simulink model "NN_MPC"  (R2018a)
settings: Solver=FixedStepAuto  SolverName=VariableStepAuto  StartTime=0.0  StopTime=40  FixedStep=0.01  RelTol=1e-3
values from neighbouring files (symbols this model uses):
  a = 0.95    [Params.mat]    (also in R_neural_function.m = 2 ./ (1 + exp(-2*n)) - 1; neural_Nc.m = 2 ./ (1 + exp(-2*n)) - 1; neural_Np.m = 2 ./ (1 + exp(-2*n)) - 1; neural_Qy.m = 2 ./ (1 + exp(-2*n)) - 1)
  Cf = 19000    [Params.mat]
  Cr = 33000    [Params.mat]
  deltau_max = 0.261799387799    [Params.mat]
  deltau_min = -0.261799387799    [Params.mat]
  dt = 0.1    [Params.mat]
  Iz = 2875    [Params.mat]
  lf = 1.2    [Params.mat]
  lr = 1.6    [Params.mat]
  m = 1575    [Params.mat]
  N = 10    [Params.mat]
  Nc = 5    [Params.mat]
  Np = 35    [Params.mat]
  Q = 5    [Params.mat]    (also in R_neural_function.m = 0; neural_Nc.m = 0; neural_Np.m = 0; neural_Qy.m = 0)
  R = 0.1    [Params.mat]
  u_max = 0.523598775598    [Params.mat]
  u_min = -0.523598775598    [Params.mat]
  y_max = 200    [Params.mat]
  y_min = -200    [Params.mat]
undefined symbols (not defined in the file or in its folder): neural_Nc, neural_Np, neural_Qy, neural_R, sigbuilder_block
libraries: autolibutils x8, autolibshared x6, vehdynlibviscommon x2, simulink x2
(part 1 of 4)
settings Model: Creator=yassine  LastModifiedBy=yassi
settings DataIOCC: ReturnWorkspaceOutputs=on
settings SFSimCC: SimUseLocalCustomCode=on
settings RTWCC: RTWUseLocalCustomCode=on

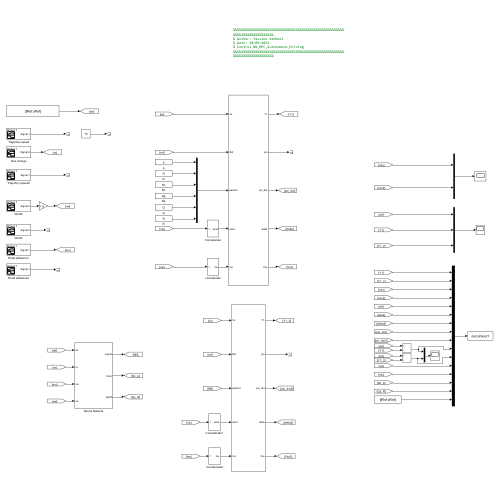
[thumbnail: Simulink's stored preview of the top-level diagram]
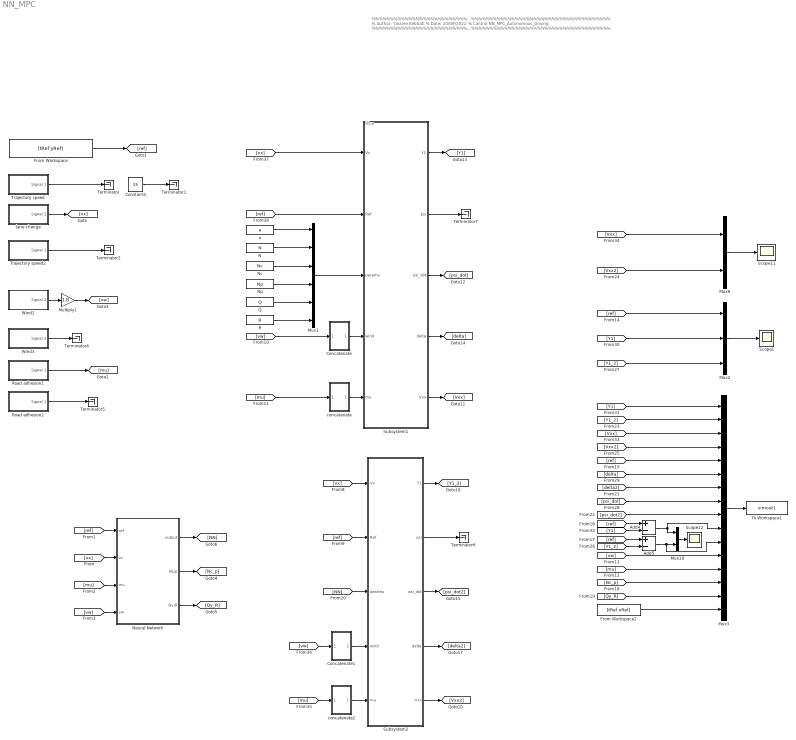
== system NN_MPC ==
  note: %%%%%%%%%%%%%%%%%%%%%%%%%%%%%%%%%%%%%%%%%%%%%%%%%%%%%%%%%%%%%%%%%%%%%%%%%%%
      | % Author: Yassine Kebbati
      | % Date: 20/09/2022
      | % Control NN_MPC_Autonomous_Driving
      | %%%%%%%%%%%%%%%%%%%%%%%%%%%%%%%%%%%%%%%%%%%%%%%%%%%%%%%%%%%%%%%%%%%%%%%%%%%
  note: Blue
  Add4 : Sum  Inputs=+-
  Add5 : Sum  Inputs=+-
  Concatenate : Subsystem
  Concatenate1 : Subsystem
  Constant4 : Constant  Value=15
  From Workspace : FromWorkspace  VariableName=[tRef yRef]
  From Workspace2 : FromWorkspace  VariableName=[tRef xRef]
  Multiply1 : Gain  Gain=1.8
  Mux1 : Mux  Inputs=6
  Mux10 : Mux  Inputs=2
  Mux2 : Mux  Inputs=3
  Mux3 : Mux  Inputs=16
  Mux9 : Mux  Inputs=2
  N : Constant  Value=N
  Nc : Constant  Value=Nc
  Neural Network : Subsystem
  Np : Constant  Value=Np
  Q : Constant  Value=Q
  R : Constant  Value=R
  Road adhesion1 : Subsystem  Tag=STV Subsys  LoadFcn=sigbuilder_block('load');  StartFcn=sigbuilder_block('start');  StopFcn=sigbuilder_block('stop');  ClipboardFcn=sigbuilder_block('clipboard');  mask(Sigbuilder block){tuvar=[0:10]}
      mask help: Simulink:masks:SigbuilderBlock_MD
      mask init:
      | if ~strcmp(get_param(bdroot(gcbh),'SimulationStatus'),'stopped') tuvar = sigbuilder_block('maskInit'); end
      settings: CopyFcn=sigbuilder_block('copy');  DeleteFcn=sigbuilder_block('delete');  ModelCloseFcn=sigbuilder_block('modelClose');  PreSaveFcn=sigbuilder_block('preSave');  PauseFcn=sigbuilder_block('pause');  ContinueFcn=sigbuilder_block('continue');  NameChangeFcn=sigbuilder_block('namechange');  OpenFcn=sigbuilder_block('open',[6 22.5 1428 689.25 ]);  CloseFcn=sigbuilder_block('close');
      mask Display: plot(0, 0, 100, 100,[2, 2, 32, 32, 2], [68, 8, 8, 68, 68],[32, 2], [38, 38], [32, 19, 2],[53, 60, 44], [32, 17, 17, 2],[16, 16, 31, 31]);txt = getActiveGroup(gcbh);text(2, 100, txt,'verticalAlignment', 'top');
  Road adhesion2 : Subsystem  Tag=STV Subsys  LoadFcn=sigbuilder_block('load');  StartFcn=sigbuilder_block('start');  StopFcn=sigbuilder_block('stop');  ClipboardFcn=sigbuilder_block('clipboard');  mask(Sigbuilder block){tuvar=[0:10]}
      mask help: Simulink:masks:SigbuilderBlock_MD
      mask init:
      | if ~strcmp(get_param(bdroot(gcbh),'SimulationStatus'),'stopped') tuvar = sigbuilder_block('maskInit'); end
      settings: CopyFcn=sigbuilder_block('copy');  DeleteFcn=sigbuilder_block('delete');  ModelCloseFcn=sigbuilder_block('modelClose');  PreSaveFcn=sigbuilder_block('preSave');  PauseFcn=sigbuilder_block('pause');  ContinueFcn=sigbuilder_block('continue');  NameChangeFcn=sigbuilder_block('namechange');  OpenFcn=sigbuilder_block('open',[1446 57 1428 689.25 ]);  CloseFcn=sigbuilder_block('close');
      mask Display: plot(0, 0, 100, 100,[2, 2, 32, 32, 2], [68, 8, 8, 68, 68],[32, 2], [38, 38], [32, 19, 2],[53, 60, 44], [32, 17, 17, 2],[16, 16, 31, 31]);txt = getActiveGroup(gcbh);text(2, 100, txt,'verticalAlignment', 'top');
  Scope1 : Scope
  Scope11 : Scope
  Scope12 : Scope
  Subsystem1 : Subsystem
  Subsystem2 : Subsystem
  Terminator{,1..2,4..7} (7 alike) : Terminator
  To Workspace1 : ToWorkspace  VariableName=simout1  SaveFormat=Timeseries  SampleTime=-1
  Trajectory speed : Subsystem  Tag=STV Subsys  LoadFcn=sigbuilder_block('load');  StartFcn=sigbuilder_block('start');  StopFcn=sigbuilder_block('stop');  ClipboardFcn=sigbuilder_block('clipboard');  mask(Sigbuilder block){tuvar=[0:10]}
      mask help: Simulink:masks:SigbuilderBlock_MD
      mask init:
      | if ~strcmp(get_param(bdroot(gcbh),'SimulationStatus'),'stopped') tuvar = sigbuilder_block('maskInit'); end
      settings: CopyFcn=sigbuilder_block('copy');  DeleteFcn=sigbuilder_block('delete');  ModelCloseFcn=sigbuilder_block('modelClose');  PreSaveFcn=sigbuilder_block('preSave');  PauseFcn=sigbuilder_block('pause');  ContinueFcn=sigbuilder_block('continue');  NameChangeFcn=sigbuilder_block('namechange');  OpenFcn=sigbuilder_block('open',[6 22.5 1428 689.25 ]);  CloseFcn=sigbuilder_block('close');
      mask Display: plot(0, 0, 100, 100,[2, 2, 32, 32, 2], [68, 8, 8, 68, 68],[32, 2], [38, 38], [32, 19, 2],[53, 60, 44], [32, 17, 17, 2],[16, 16, 31, 31]);txt = getActiveGroup(gcbh);text(2, 100, txt,'verticalAlignment', 'top');
  Trajectory speed2 : Subsystem  Tag=STV Subsys  LoadFcn=sigbuilder_block('load');  StartFcn=sigbuilder_block('start');  StopFcn=sigbuilder_block('stop');  ClipboardFcn=sigbuilder_block('clipboard');  mask(Sigbuilder block){tuvar=[0:10]}
      mask help: Simulink:masks:SigbuilderBlock_MD
      mask init:
      | if ~strcmp(get_param(bdroot(gcbh),'SimulationStatus'),'stopped') tuvar = sigbuilder_block('maskInit'); end
      settings: CopyFcn=sigbuilder_block('copy');  DeleteFcn=sigbuilder_block('delete');  ModelCloseFcn=sigbuilder_block('modelClose');  PreSaveFcn=sigbuilder_block('preSave');  PauseFcn=sigbuilder_block('pause');  ContinueFcn=sigbuilder_block('continue');  NameChangeFcn=sigbuilder_block('namechange');  OpenFcn=sigbuilder_block('open',[6 3.75 1428 648.75 ]);  CloseFcn=sigbuilder_block('close');
      mask Display: plot(0, 0, 100, 100,[2, 2, 32, 32, 2], [68, 8, 8, 68, 68],[32, 2], [38, 38], [32, 19, 2],[53, 60, 44], [32, 17, 17, 2],[16, 16, 31, 31]);txt = getActiveGroup(gcbh);text(2, 100, txt,'verticalAlignment', 'top');
  Wind2 : Subsystem  Tag=STV Subsys  LoadFcn=sigbuilder_block('load');  StartFcn=sigbuilder_block('start');  StopFcn=sigbuilder_block('stop');  ClipboardFcn=sigbuilder_block('clipboard');  mask(Sigbuilder block){tuvar=[0:10]}
      mask help: Simulink:masks:SigbuilderBlock_MD
      mask init:
      | if ~strcmp(get_param(bdroot(gcbh),'SimulationStatus'),'stopped') tuvar = sigbuilder_block('maskInit'); end
      settings: CopyFcn=sigbuilder_block('copy');  DeleteFcn=sigbuilder_block('delete');  ModelCloseFcn=sigbuilder_block('modelClose');  PreSaveFcn=sigbuilder_block('preSave');  PauseFcn=sigbuilder_block('pause');  ContinueFcn=sigbuilder_block('continue');  NameChangeFcn=sigbuilder_block('namechange');  OpenFcn=sigbuilder_block('open',[6 85.5 1428 608.25 ]);  CloseFcn=sigbuilder_block('close');
      mask Display: plot(0, 0, 100, 100,[2, 2, 32, 32, 2], [68, 8, 8, 68, 68],[32, 2], [38, 38], [32, 19, 2],[53, 60, 44], [32, 17, 17, 2],[16, 16, 31, 31]);txt = getActiveGroup(gcbh);text(2, 100, txt,'verticalAlignment', 'top');
  Wind3 : Subsystem  Tag=STV Subsys  LoadFcn=sigbuilder_block('load');  StartFcn=sigbuilder_block('start');  StopFcn=sigbuilder_block('stop');  ClipboardFcn=sigbuilder_block('clipboard');  mask(Sigbuilder block){tuvar=[0:10]}
      mask help: Simulink:masks:SigbuilderBlock_MD
      mask init:
      | if ~strcmp(get_param(bdroot(gcbh),'SimulationStatus'),'stopped') tuvar = sigbuilder_block('maskInit'); end
      settings: CopyFcn=sigbuilder_block('copy');  DeleteFcn=sigbuilder_block('delete');  ModelCloseFcn=sigbuilder_block('modelClose');  PreSaveFcn=sigbuilder_block('preSave');  PauseFcn=sigbuilder_block('pause');  ContinueFcn=sigbuilder_block('continue');  NameChangeFcn=sigbuilder_block('namechange');  OpenFcn=sigbuilder_block('open',[6 22.5 1428 689.25 ]);  CloseFcn=sigbuilder_block('close');
      mask Display: plot(0, 0, 100, 100,[2, 2, 32, 32, 2], [68, 8, 8, 68, 68],[32, 2], [38, 38], [32, 19, 2],[53, 60, 44], [32, 17, 17, 2],[16, 16, 31, 31]);txt = getActiveGroup(gcbh);text(2, 100, txt,'verticalAlignment', 'top');
  a : Constant  Value=a
  concatenate : Subsystem
  concatenate2 : Subsystem
  lane change : Subsystem  Tag=STV Subsys  LoadFcn=sigbuilder_block('load');  StartFcn=sigbuilder_block('start');  StopFcn=sigbuilder_block('stop');  ClipboardFcn=sigbuilder_block('clipboard');  mask(Sigbuilder block){tuvar=[0:10]}
      mask help: Simulink:masks:SigbuilderBlock_MD
      mask init:
      | if ~strcmp(get_param(bdroot(gcbh),'SimulationStatus'),'stopped') tuvar = sigbuilder_block('maskInit'); end
      settings: CopyFcn=sigbuilder_block('copy');  DeleteFcn=sigbuilder_block('delete');  ModelCloseFcn=sigbuilder_block('modelClose');  PreSaveFcn=sigbuilder_block('preSave');  PauseFcn=sigbuilder_block('pause');  ContinueFcn=sigbuilder_block('continue');  NameChangeFcn=sigbuilder_block('namechange');  OpenFcn=sigbuilder_block('open',[6 22.5 1428 689.25 ]);  CloseFcn=sigbuilder_block('close');
      mask Display: plot(0, 0, 100, 100,[2, 2, 32, 32, 2], [68, 8, 8, 68, 68],[32, 2], [38, 38], [32, 19, 2],[53, 60, 44], [32, 17, 17, 2],[16, 16, 31, 31]);txt = getActiveGroup(gcbh);text(2, 100, txt,'verticalAlignment', 'top');
  wires:
  Neural Network/2(Nc/p) -> [Nc_p]
  [vw] -> Neural Network/4(vw)
  [mu] -> Neural Network/3(mu)
  Neural Network/1(output) -> [NN]
  Neural Network/3(Qy/R) -> [Qy_R]
  [ref] -> Neural Network/1(ref)
  [vx] -> Neural Network/2(vx)
  Subsystem1/5(Vxx) -> [Vxx]
  Q/1 -> Mux1/5
  [Nc_p] -> Mux3/14
  Subsystem1/2(psi) -> Terminator7/1
  [vw] -> Concatenate/1(In1)
  [NN] -> Subsystem2/3(params)
  Subsystem1/4(delta) -> [delta]
  R/1 -> Mux1/6
  [Y1_2] -> Mux2/3
  [Y1] -> Add4/2
  Subsystem1/1(Y1) -> [Y1]
  Subsystem2/2(psi) -> Terminator6/1
  [psi_dot2] -> Mux3/9
  Np/1 -> Mux1/4
  [Vxx] -> Mux3/3
  [psi_dot] -> Mux3/8
  [mu] -> concatenate2/1(In1)
  lane change/1(Signal 2) -> [vx]
  Trajectory speed2/1(Signal 1) -> Terminator2/1
  [vx] -> Subsystem2/1(Vx)
  From Workspace/1 -> [ref]
  [Qy_R] -> Mux3/15
  Road adhesion2/1(Signal 1) -> Terminator5/1
  concatenate/1(mu) -> Subsystem1/5(mu)
  Mux9/1 -> Scope11/1
  Wind2/1(Signal 2) -> Multiply1/1
  From Workspace2/1 -> Mux3/16
  Add4/1 -> Mux3/10, Mux10/1
  Trajectory speed/1(Signal 1) -> Terminator/1
  [ref] -> Add5/1
  [ref] -> Subsystem1/2("Ref ")
  Concatenate1/1(wind) -> Subsystem2/4(wind)
  [ref] -> Subsystem2/2("Ref ")
  [vw] -> Concatenate1/1(In1)
  [Y1] -> Mux2/2
  Add5/1 -> Mux3/11, Mux10/2
  [delta] -> Mux3/6
  Nc/1 -> Mux1/3
  [Y1_2] -> Add5/2
  [Vxx2] -> Mux9/2
  Mux3/1 -> To Workspace1/1
  Mux2/1 -> Scope1/1
  Concatenate/1(wind) -> Subsystem1/4(wind)
  [Y1_2] -> Mux3/2
  [Vxx2] -> Mux3/4
  Subsystem1/3(psi_dot) -> [psi_dot]
  Subsystem2/1(Y1) -> [Y1_2]
  Wind3/1(Signal 2) -> Terminator4/1
  Subsystem2/5(Vxx) -> [Vxx2]
  [delta2] -> Mux3/7
  [ref] -> Mux3/5
  Subsystem2/4(delta) -> [delta2]
  Mux1/1 -> Subsystem1/3(params)
  Multiply1/1 -> [vw]
  Road adhesion1/1(Signal 1) -> [mu]
  Constant4/1 -> Terminator1/1
  [Vxx] -> Mux9/1
  Mux10/1 -> Scope12/1
  [ref] -> Mux2/1
  concatenate2/1(mu) -> Subsystem2/5(mu)
  [mu] -> Mux3/13
  [mu] -> concatenate/1(In1)
  [Y1] -> Mux3/1
  [vw] -> Mux3/12
  Subsystem2/3(psi_dot) -> [psi_dot2]
  [vx] -> Subsystem1/1(Vx)
  N/1 -> Mux1/2
  a/1 -> Mux1/1
  [ref] -> Add4/1

== system NN_MPC/Concatenate ==
  In1 : Inport
  Constant1 : Constant  Value=0
  Matrix Concatenate : Concatenate  NumInputs=3  Mode=Multidimensional array  ConcatenateDimension=2
  wind : Outport
  wires:
  Constant1/1 -> Matrix Concatenate/3, Matrix Concatenate/1
  In1/1 -> Matrix Concatenate/2
  Matrix Concatenate/1 -> wind/1

== system NN_MPC/Concatenate1 ==
  In1 : Inport
  Constant1 : Constant  Value=0
  Matrix Concatenate : Concatenate  NumInputs=3  Mode=Multidimensional array  ConcatenateDimension=2
  wind : Outport
  wires:
  Constant1/1 -> Matrix Concatenate/3, Matrix Concatenate/1
  In1/1 -> Matrix Concatenate/2
  Matrix Concatenate/1 -> wind/1

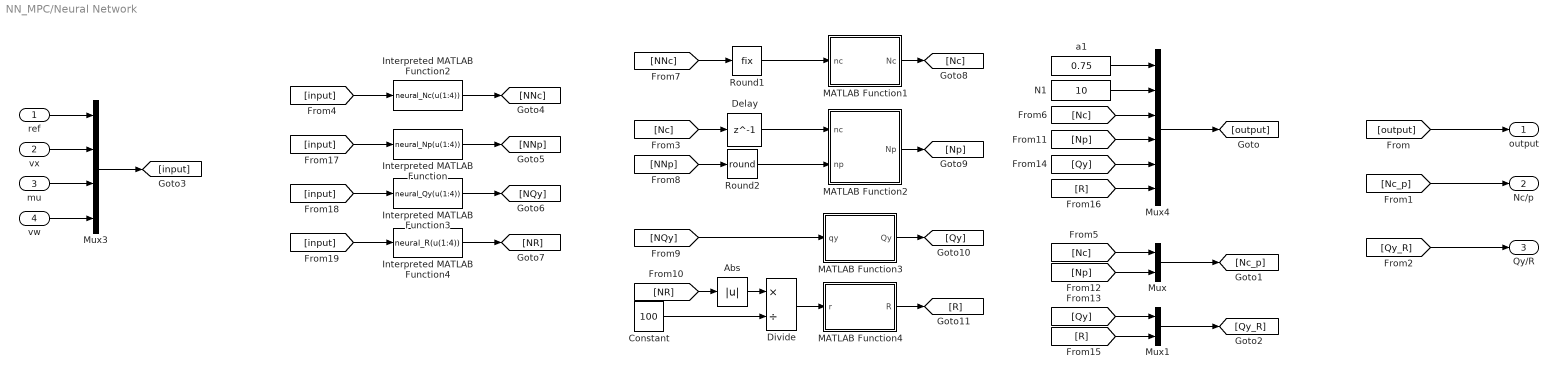
== system NN_MPC/Neural Network ==
  ref : Inport
  vx : Inport  Port=2
  mu : Inport  Port=3
  vw : Inport  Port=4
  Abs : Abs
  Constant : Constant  Value=100
  Delay : Delay  DelayLength=1
  Divide : Product  Inputs=*/
  Interpreted MATLAB Function : MATLABFcn  MATLABFcn=neural_Np(u(1:4))
  Interpreted MATLAB Function2 : MATLABFcn  MATLABFcn=neural_Nc(u(1:4))
  Interpreted MATLAB Function3 : MATLABFcn  MATLABFcn=neural_Qy(u(1:4))
  Interpreted MATLAB Function4 : MATLABFcn  MATLABFcn=neural_R(u(1:4))
  MATLAB Function1 : MATLAB Function  TreatAsAtomicUnit=on
  MATLAB Function2 : MATLAB Function  TreatAsAtomicUnit=on
  MATLAB Function3 : MATLAB Function  TreatAsAtomicUnit=on
  MATLAB Function4 : MATLAB Function  TreatAsAtomicUnit=on
  Mux : Mux  Inputs=2
  Mux1 : Mux  Inputs=2
  Mux3 : Mux
  Mux4 : Mux  Inputs=6
  N1 : Constant  Value=10
  Round1 : Rounding  Operator=fix
  Round2 : Rounding  Operator=round
  a1 : Constant  Value=0.75
  output : Outport
  Nc/p : Outport  Port=2
  Qy/R : Outport  Port=3
  wires:
  [NQy] -> MATLAB Function3/1(qy)
  [NNp] -> Round2/1
  [output] -> output/1
  [Nc] -> Delay/1
  Delay/1 -> MATLAB Function2/1(nc)
  ref/1 -> Mux3/1
  [NNc] -> Round1/1
  vx/1 -> Mux3/2
  [NR] -> Abs/1
  Round1/1 -> MATLAB Function1/1(nc)
  Round2/1 -> MATLAB Function2/2(np)
  Abs/1 -> Divide/1
  mu/1 -> Mux3/3
  vw/1 -> Mux3/4
  Divide/1 -> MATLAB Function4/1(r)
  Constant/1 -> Divide/2
  N1/1 -> Mux4/2
  a1/1 -> Mux4/1
  Mux/1 -> [Nc_p]
  Mux1/1 -> [Qy_R]
  Mux4/1 -> [output]
  [Nc_p] -> Nc/p/1
  [Qy_R] -> Qy/R/1
  Mux3/1 -> [input]
  [input] -> Interpreted MATLAB Function2/1
  [input] -> Interpreted MATLAB Function/1
  [input] -> Interpreted MATLAB Function3/1
  [input] -> Interpreted MATLAB Function4/1
  Interpreted MATLAB Function2/1 -> [NNc]
  Interpreted MATLAB Function/1 -> [NNp]
  Interpreted MATLAB Function3/1 -> [NQy]
  Interpreted MATLAB Function4/1 -> [NR]
  MATLAB Function1/1(Nc) -> [Nc]
  [Nc] -> Mux/1
  [Nc] -> Mux4/3
  MATLAB Function2/1(Np) -> [Np]
  [Np] -> Mux4/4
  [Np] -> Mux/2
  MATLAB Function3/1(Qy) -> [Qy]
  [Qy] -> Mux1/1
  [Qy] -> Mux4/5
  MATLAB Function4/1(R) -> [R]
  [R] -> Mux4/6
  [R] -> Mux1/2

== system NN_MPC/Road adhesion1 ==
  Demux : Demux  Tag=STV Demux  Outputs=1
      settings: DisplayOption=none
  FromWs : FromWorkspace  Tag=STV FromWs  VariableName=tuvar
      SigBuilderData=|
      | common.afterFinalStr = 'Extrapolate'
      | common.sampleTime = 0
      | dataSet.timeRange = [0 28]
      | dataSet.name = 'Group 1'
      | sbobj.Groups.Name = 'Group 1'
      | sbobj.Groups.Signals.Name = 'Signal 1'
      | sbobj.Groups.Signals.XData = [0 0.1 0.2 0.3 0.4 0.5 0.6 0.7 0.8 0.9 1 1.1 1.2 1.3 1.4 1.5 1.6 1.7 1.8 1.9 2 2.1 2.2 2.3 2.4 2.5 2.6 2.7 2.8 2.9 3 3.1 3.2 3.3 3.4 3.5 3.6 3.7 3.8 3.9 4 4.1 4.2 4.3 4.4 4.5 4.6 4.7 4.8 4.9 5 5.1 5.2 5.3 5.4 5.5 5.6 5.7 5.8 5.9 6 6.1 6.2 6.3 6.4 6.5 6.6 6.7 6.8 6.9 7 7.1 7.2 7.3 7.4 7.5 7.6 7.7 7.8 7.9 8 8.1 8.2 8.3 8.4 8.5 8.6 8.6 8.7 8.7 8.8 8.8 8.9 8.9 9 9.1 9.2 9.3 9.4 9.5 9.6 9.7 9.8 9.9 10 10.1 10.2 10.3 10.4 10.5 10.6 10.7 10.8 10.9 11 11.1 11.2 11.3 11.4 11.5 11.6 11.7 11.8 11.9 12 12.1 12.2 12.3 12.4 12.5 12.6 12.7 12.8 12.9 13 13.1 13.2 13.3 13.4 13.5 13.6 13.7 13.8 13.9 14 14.1 14.2 14.3 14.4 14.5 14.6 14.7 14.8 14.9 15 15.1 15.2 15.2 15.3 15.4 15.5 15.6 15.7 15.8 15.9 16 16.1 16.2 16.3 16.4 16.5 16.6 16.7 16.8 16.9 17 17.1 17.2 17.3 17.4 17.5 17.6 17.7 17.8 17.9 18 18.1 18.2 18.3 18.4 18.5 18.6 18.7 18.8 18.9 19 19.1 19.2 19.3 19.4 19.5 19.6 19.7 19.8 19.9 20 20.1 20.2 20.3 20.4 20.5 20.6 20.7 20.8 20.9 21 21.1 21.2 21.3 21.4 21.5 21.6 21.7 21.8 21.9 22 22.1 22.2 22.3 22.4 22.5 22.6 22.7 22.8 22.9 23 23.1 23.2 23.3 23.4 23.5 23.6 23.7 23.8 23.9 24 24.1 24.2 24.3 24.4 24.5 24.6 24.7 24.8 24.9 25 25.1 25.2 25.3 25.4 25.5 25.6 25.7 25.8 25.9 26 26.1 26.2 26.3 26.4 26.5 26.6 26.7 26.8 28]
      | sbobj.Groups.Signals.YData = [0.9 0.9 0.9 0.9 0.9 0.9 0.9 0.9 0.9 0.9 0.9 0.9 0.9 0.9 0.9 0.9 0.9 0.9 0.9 0.9 0.9 0.9 0.899 0.896 0.892 0.888 0.883 0.88 0.876 0.866 0.846 0.806 0.781 0.767 0.754 0.739 0.721 0.714 0.703 0.704 0.713 0.725 0.735 0.745 0.756 0.758 0.759 0.761 0.762 0.759 0.756 0.751 0.749 0.751 0.756 0.765 0.771 0.78 0.789 0.796 0.802 0.805 0.804 0.801 0.798 0.795 0.792 0.789 0.786 0.783 0.78 0.774 0.77 0.767 0.768 0.767 0.766 0.763 0.762 0.761 0.757 0.753 0.739 0.711 0.689 0.657 0.634 0.633 0.623 0.624 0.614 0.615 0.613 0.612 0.615 0.618 0.619 0.625 0.721 0.728 0.732 0.737 0.75 0.759 0.779 0.79 0.798 0.804 0.814 0.814 0.821 0.825 0.825 0.821 0.831 0.838 0.848 0.848 0.849 0.841 0.825 0.805 0.782 0.771 0.768 0.755 0.749 0.735 0.714 0.708 0.702 0.696 0.69 0.684 0.678 0.672 0.666 0.66 0.654 0.648 0.642 0.636 0.63 0.624 0.618 0.612 0.606 0.6 0.596 0.594 0.591 0.588 0.586 0.585 0.576 0.569 0.542 0.541 0.535 0.518 0.506 0.504 0.504 0.501 0.501 0.502 0.504 0.505 0.504 0.504 0.504 0.504 0.502 0.502 0.503 0.503 0.514 0.519 0.527 0.528 0.53 0.529 0.524 0.523 0.527 0.535 0.549 0.55 0.554 0.55 0.547 0.55 0.561 0.577 0.58 0.582 0.585 0.588 0.593 0.591 0.583 0.571 0.559 0.554 0.573 0.589 0.607 0.628 0.643 0.66 0.67 0.671 0.672 0.686 0.701 0.717 0.736 0.744 0.752 0.76 0.768 0.776 0.78 0.786 0.788 0.788 0.789 0.79 0.798 0.807 0.814 0.825 0.834 0.849 0.856 0.863 0.865 0.868 0.861 0.843 0.829 0.811 0.805 0.8 0.8 0.8 0.8 0.8 0.8 0.8 0.8 0.8 0.8 0.8 0.8 0.8 0.8 0.8 0.8 0.8 0.8 0.8 0.8 0.8 0.8 0.8 0.8 0.8 0.8 0.8 0.8 0.8 0.8 0.8 0.8]
      | sbobj.Groups.TimeRange = [0 28]
  Signal 1 : Outport  Tag=STV Outport
  wires:
  FromWs/1 -> Demux/1
  Demux/1 -> Signal 1/1

== system NN_MPC/Road adhesion2 ==
  Demux : Demux  Tag=STV Demux  Outputs=1
      settings: DisplayOption=none
  FromWs : FromWorkspace  Tag=STV FromWs  VariableName=tuvar
      SigBuilderData=|
      | common.afterFinalStr = 'Extrapolate'
      | common.sampleTime = 0
      | dataSet.timeRange = [0 200]
      | dataSet.name = 'Group 1'
      | sbobj.Groups.Name = 'Group 1'
      | sbobj.Groups.Signals.Name = 'Signal 1'
      | sbobj.Groups.Signals.XData = [0 1 2 3 4 5 6 7 8 9 10 11 12 13 14 15 16 17 18 19 20 21 22 23 24 25 26 27 28 29 30 31 32 33 34 35 36 37 38 39 40 40 41 41 42 43 44 45 46 47 48 49 50 51 52 53 54 55 56 57 58 59 60 61 62 63 64 65 66 67 68 69 70 71 72 73 74 75 76 77 78 79 80 81 82 83 84 85 86 87 88 89 90 91 92 93 94 95 96 97 98 99 100 101 102 103 104 105 106 107 108 109 110 111 112 113 114 115 116 117 118 119 120 121 122 123 124 125 126 127 128 129 130 131 132 133 134 135 136 137 138 139 140 141 142 143 144 145 146 147 148 149 150 151 152 153 154 155 156 157 158 159 160 161 162 163 164 165 166 167 168 169 170 171 172 173 174 175 176 177 178 179 180 181 182 183 184 185 186 187 188 189 190 191 192 193 194 195 196 197 198 199 200]
      | sbobj.Groups.Signals.YData = [0.95 0.94 0.93 0.92 0.91 0.9 0.89 0.88 0.87 0.86 0.85 0.84 0.83 0.82 0.81 0.8 0.79 0.78 0.77 0.76 0.75 0.74 0.739 0.733 0.726 0.733 0.728 0.719 0.688 0.669 0.662 0.65 0.654 0.662 0.66 0.659 0.659 0.665 0.664 0.666 0.666 0.665 0.665 0.666 0.664 0.658 0.652 0.653 0.65 0.645 0.641 0.635 0.631 0.63 0.629 0.628 0.627 0.626 0.625 0.624 0.623 0.622 0.621 0.62 0.619 0.618 0.617 0.616 0.615 0.614 0.613 0.612 0.611 0.61 0.609 0.608 0.607 0.606 0.605 0.604 0.603 0.602 0.601 0.6 0.6 0.602 0.604 0.606 0.608 0.61 0.612 0.614 0.616 0.618 0.62 0.622 0.624 0.626 0.628 0.63 0.632 0.634 0.636 0.638 0.64 0.64 0.65 0.66 0.67 0.68 0.69 0.7 0.71 0.72 0.73 0.74 0.75 0.76 0.77 0.78 0.79 0.8 0.81 0.82 0.82 0.825 0.83 0.835 0.84 0.845 0.85 0.85 0.844 0.838 0.832 0.826 0.82 0.814 0.81 0.79 0.77 0.75 0.73 0.71 0.69 0.67 0.65 0.63 0.61 0.59 0.58 0.578 0.576 0.574 0.572 0.57 0.568 0.566 0.564 0.562 0.56 0.558 0.556 0.554 0.552 0.55 0.55 0.58 0.61 0.64 0.67 0.7 0.73 0.75 0.755 0.76 0.765 0.77 0.775 0.78 0.785 0.79 0.795 0.8 0.8 0.81 0.82 0.83 0.84 0.85 0.86 0.87 0.88 0.89 0.9 0.91 0.92 0.93 0.94 0.95 0.955 0.96 0.96]
      | sbobj.Groups.TimeRange = [0 200]
  Signal 1 : Outport  Tag=STV Outport
  wires:
  FromWs/1 -> Demux/1
  Demux/1 -> Signal 1/1

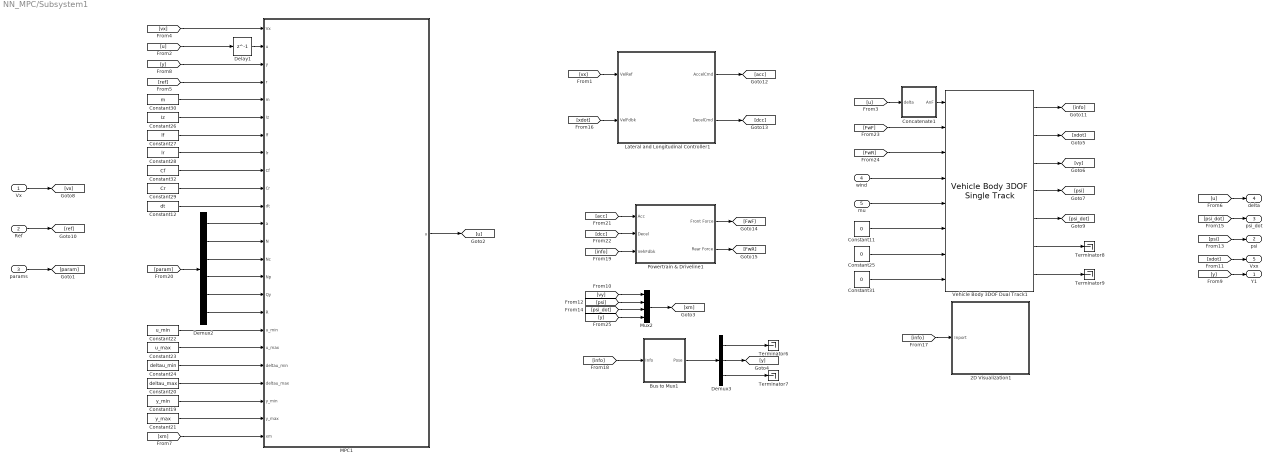
== system NN_MPC/Subsystem1 ==
  Vx : Inport
  "Ref " : Inport  Port=2
  params : Inport  Port=3
  wind : Inport  Port=4
  mu : Inport  Port=5
  2D Visualization1 : Subsystem
      mask Display: image("visualization.JPG");
  Bus to Mux1 : Subsystem
  Concatenate1 : Subsystem
  Constant11 : Constant  Value=0
  Constant12 : Constant  Value=dt
  Constant19 : Constant  Value=y_min
  Constant20 : Constant  Value=deltau_max
  Constant21 : Constant  Value=y_max
  Constant22 : Constant  Value=u_min
  Constant23 : Constant  Value=u_max
  Constant24 : Constant  Value=deltau_min
  Constant25 : Constant  Value=0
  Constant26 : Constant  Value=Iz
  Constant27 : Constant  Value=lf
  Constant28 : Constant  Value=lr
  Constant29 : Constant  Value=Cr
  Constant30 : Constant  Value=m
  Constant31 : Constant  Value=0
  Constant32 : Constant  Value=Cf
  Delay1 : Delay  DelayLength=1
  Demux2 : Demux  Outputs=6
  Demux3 : Demux  Outputs=3
  Lateral and Longitudinal Controller1 : Subsystem
  MPC1 : MATLAB Function  TreatAsAtomicUnit=on
  Mux2 : Mux
  Powertrain & Driveline1 : Subsystem
      mask Display: image('vdbslibpt.png');
  Terminator{6..9} (4 alike) : Terminator
  Vehicle Body 3DOF Dual Track1 : autolibshared/Vehicle Body 3DOF Single Track  trackMode=Dual  inputMode=External longitudinal forces  frontSteerMode=on  rearSteerMode=off  windMode=on  muMode=on  extFMode=off  extMMode=off  htchFMode=off  htchMMode=off  aMode=2  NF=2  NR=2  m=1575  a=1.2  b=1.6  h=0.35  dh=1  hh=0.2  X_o=0  xdot_o=0  CalphaMode=off  sigmaMode=on  hl=0  w=[1.4,1.4]  Cy_f=19e3  Cy_r=33e3  sigma_f=.1  sigma_r=.1  alpha_f_brk=[-.1 .1]  Cy_f_data=[-9e3 9e3]  alpha_r_brk=[-.1 .1]  Cy_r_data=[-9e3 9e3]  Y_o=0  ydot_o=0  Izz=2875  psi_o=0  r_o=0  Af=2  Cd=.3  Cl=.1  Cpm=.1  beta_w=[0:0.01:0.3]  Cs=[0:0.03:0.9]  Cym=[0:0.01:0.3]  Pabs=101325  Tair=273  g=9.81  mu=1  xdot_tol=0.01  Fznom=5000  Fxtire_sat=7e4  Fytire_sat=7e4
  Y1 : Outport
  psi : Outport  Port=2
  psi_dot : Outport  Port=3
  delta : Outport  Port=4
  Vxx : Outport  Port=5
  wires:
  [vy] -> Mux2/1
  [psi] -> Mux2/2
  Vehicle Body 3DOF Dual Track1/1 -> [info]
  [FwF] -> Vehicle Body 3DOF Dual Track1/2
  [u] -> Concatenate1/1(delta)
  Demux3/2 -> [y]
  [vx] -> Lateral and Longitudinal Controller1/1(VelRef)
  Concatenate1/1(AnF) -> Vehicle Body 3DOF Dual Track1/1
  Constant27/1 -> MPC1/7(lf)
  Constant30/1 -> MPC1/5(m)
  Lateral and Longitudinal Controller1/1(AccelCmd) -> [acc]
  Demux2/3 -> MPC1/14(Nc)
  Demux2/5 -> MPC1/16(Qy)
  Demux3/1 -> Terminator6/1
  Demux3/3 -> Terminator7/1
  Constant20/1 -> MPC1/21(deltau_max)
  Constant25/1 -> Vehicle Body 3DOF Dual Track1/7
  Constant21/1 -> MPC1/23(y_max)
  Constant24/1 -> MPC1/20(deltau_min)
  Constant23/1 -> MPC1/19(u_max)
  Vehicle Body 3DOF Dual Track1/7 -> Terminator9/1
  Constant29/1 -> MPC1/10(Cr)
  mu/1 -> Vehicle Body 3DOF Dual Track1/5
  Constant32/1 -> MPC1/9(Cf)
  Constant22/1 -> MPC1/18(u_min)
  Constant26/1 -> MPC1/6(Iz)
  wind/1 -> Vehicle Body 3DOF Dual Track1/4
  Vehicle Body 3DOF Dual Track1/2 -> [xdot]
  Vehicle Body 3DOF Dual Track1/6 -> Terminator8/1
  Demux2/2 -> MPC1/13(N)
  [info] -> Bus to Mux1/1(Info)
  Constant31/1 -> Vehicle Body 3DOF Dual Track1/8
  [u] -> Delay1/1
  [vx] -> MPC1/1(Vx)
  "Ref "/1 -> [ref]
  [info] -> Powertrain & Driveline1/3(VehFdbk)
  Constant19/1 -> MPC1/22(y_min)
  [info] -> 2D Visualization1/1(Inport)
  Vehicle Body 3DOF Dual Track1/4 -> [psi]
  Vx/1 -> [vx]
  Demux2/6 -> MPC1/17(R)
  Constant28/1 -> MPC1/8(lr)
  [y] -> Y1/1
  Constant12/1 -> MPC1/11(dt)
  [acc] -> Powertrain & Driveline1/1(Acc)
  [psi] -> psi/1
  [xdot] -> Vxx/1
  Bus to Mux1/1(Pose) -> Demux3/1
  [xdot] -> Lateral and Longitudinal Controller1/2(VelFdbk)
  Powertrain & Driveline1/2(Rear Force) -> [FwR]
  Vehicle Body 3DOF Dual Track1/5 -> [psi_dot]
  [y] -> Mux2/4
  Mux2/1 -> [xm]
  Delay1/1 -> MPC1/2("u ")
  params/1 -> [param]
  Constant11/1 -> Vehicle Body 3DOF Dual Track1/6
  [FwR] -> Vehicle Body 3DOF Dual Track1/3
  [y] -> MPC1/3(y)
  [u] -> delta/1
  MPC1/1(u) -> [u]
  [param] -> Demux2/1
  Lateral and Longitudinal Controller1/2(DecelCmd) -> [dcc]
  [dcc] -> Powertrain & Driveline1/2(Decel)
  [ref] -> MPC1/4(r)
  Vehicle Body 3DOF Dual Track1/3 -> [vy]
  Demux2/1 -> MPC1/12(a)
  Powertrain & Driveline1/1(Front Force) -> [FwF]
  [psi_dot] -> Mux2/3
  Demux2/4 -> MPC1/15(Np)
  [xm] -> MPC1/24(xm)
  [psi_dot] -> psi_dot/1

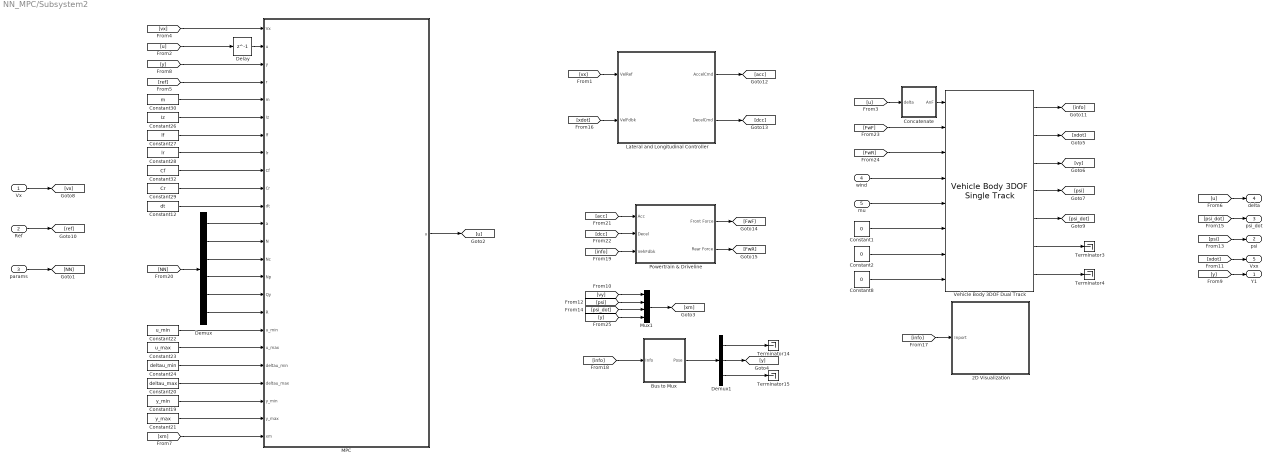
== system NN_MPC/Subsystem2 ==
  Vx : Inport
  "Ref " : Inport  Port=2
  params : Inport  Port=3
  wind : Inport  Port=4
  mu : Inport  Port=5
  2D Visualization : Subsystem
      mask Display: image("visualization.JPG");
  Bus to Mux : Subsystem
  Concatenate : Subsystem
  Constant1 : Constant  Value=0
  Constant12 : Constant  Value=dt
  Constant19 : Constant  Value=y_min
  Constant2 : Constant  Value=0
  Constant20 : Constant  Value=deltau_max
  Constant21 : Constant  Value=y_max
  Constant22 : Constant  Value=u_min
  Constant23 : Constant  Value=u_max
  Constant24 : Constant  Value=deltau_min
  Constant26 : Constant  Value=Iz
  Constant27 : Constant  Value=lf
  Constant28 : Constant  Value=lr
  Constant29 : Constant  Value=Cr
  Constant30 : Constant  Value=m
  Constant32 : Constant  Value=Cf
  Constant8 : Constant  Value=0
  Delay : Delay  DelayLength=1
  Demux : Demux  Outputs=6
  Demux1 : Demux  Outputs=3
  Lateral and Longitudinal Controller : Subsystem
  MPC : MATLAB Function  TreatAsAtomicUnit=on
  Mux1 : Mux
  Powertrain & Driveline : Subsystem
      mask Display: image('vdbslibpt.png');
  Terminator{3..4,14..15} (4 alike) : Terminator
  Vehicle Body 3DOF Dual Track : autolibshared/Vehicle Body 3DOF Single Track  trackMode=Dual  inputMode=External longitudinal forces  frontSteerMode=on  rearSteerMode=off  windMode=on  muMode=on  extFMode=off  extMMode=off  htchFMode=off  htchMMode=off  aMode=2  NF=2  NR=2  m=1575  a=1.2  b=1.6  h=0.35  dh=1  hh=0.2  X_o=0  xdot_o=0  CalphaMode=off  sigmaMode=on  hl=0  w=[1.4,1.4]  Cy_f=19e3  Cy_r=33e3  sigma_f=.1  sigma_r=.1  alpha_f_brk=[-.1 .1]  Cy_f_data=[-9e3 9e3]  alpha_r_brk=[-.1 .1]  Cy_r_data=[-9e3 9e3]  Y_o=0  ydot_o=0  Izz=2875  psi_o=0  r_o=0  Af=2  Cd=.3  Cl=.1  Cpm=.1  beta_w=[0:0.01:0.3]  Cs=[0:0.03:0.9]  Cym=[0:0.01:0.3]  Pabs=101325  Tair=273  g=9.81  mu=1  xdot_tol=0.01  Fznom=5000  Fxtire_sat=7e4  Fytire_sat=7e4
  Y1 : Outport
  psi : Outport  Port=2
  psi_dot : Outport  Port=3
  delta : Outport  Port=4
  Vxx : Outport  Port=5
  wires:
  Demux/2 -> MPC/13(N)
  Bus to Mux/1(Pose) -> Demux1/1
  [info] -> 2D Visualization/1(Inport)
  Constant8/1 -> Vehicle Body 3DOF Dual Track/8
  Powertrain & Driveline/1(Front Force) -> [FwF]
  [vx] -> MPC/1(Vx)
  Demux/6 -> MPC/17(R)
  Vehicle Body 3DOF Dual Track/7 -> Terminator4/1
  Constant29/1 -> MPC/10(Cr)
  Demux/5 -> MPC/16(Qy)
  Vehicle Body 3DOF Dual Track/2 -> [xdot]
  Demux/1 -> MPC/12(a)
  [acc] -> Powertrain & Driveline/1(Acc)
  Powertrain & Driveline/2(Rear Force) -> [FwR]
  Constant1/1 -> Vehicle Body 3DOF Dual Track/6
  [dcc] -> Powertrain & Driveline/2(Decel)
  Constant2/1 -> Vehicle Body 3DOF Dual Track/7
  Constant24/1 -> MPC/20(deltau_min)
  Constant32/1 -> MPC/9(Cf)
  Delay/1 -> MPC/2("u ")
  Demux/4 -> MPC/15(Np)
  Constant27/1 -> MPC/7(lf)
  Constant20/1 -> MPC/21(deltau_max)
  Mux1/1 -> [xm]
  Constant30/1 -> MPC/5(m)
  Demux1/1 -> Terminator14/1
  Constant28/1 -> MPC/8(lr)
  Constant21/1 -> MPC/23(y_max)
  Demux1/3 -> Terminator15/1
  Demux/3 -> MPC/14(Nc)
  [ref] -> MPC/4(r)
  Constant12/1 -> MPC/11(dt)
  Constant22/1 -> MPC/18(u_min)
  Constant23/1 -> MPC/19(u_max)
  [u] -> Delay/1
  Vehicle Body 3DOF Dual Track/6 -> Terminator3/1
  Concatenate/1(AnF) -> Vehicle Body 3DOF Dual Track/1
  Constant19/1 -> MPC/22(y_min)
  Constant26/1 -> MPC/6(Iz)
  [NN] -> Demux/1
  wind/1 -> Vehicle Body 3DOF Dual Track/4
  mu/1 -> Vehicle Body 3DOF Dual Track/5
  Vx/1 -> [vx]
  "Ref "/1 -> [ref]
  params/1 -> [NN]
  [vx] -> Lateral and Longitudinal Controller/1(VelRef)
  MPC/1(u) -> [u]
  [u] -> Concatenate/1(delta)
  [u] -> delta/1
  [xm] -> MPC/24(xm)
  [y] -> MPC/3(y)
  Demux1/2 -> [y]
  [y] -> Y1/1
  [xdot] -> Lateral and Longitudinal Controller/2(VelFdbk)
  [xdot] -> Vxx/1
  Vehicle Body 3DOF Dual Track/3 -> [vy]
  [vy] -> Mux1/1
  [psi] -> Mux1/2
  Vehicle Body 3DOF Dual Track/4 -> [psi]
  [psi] -> psi/1
  [psi_dot] -> Mux1/3
  Vehicle Body 3DOF Dual Track/5 -> [psi_dot]
  [psi_dot] -> psi_dot/1
  [info] -> Bus to Mux/1(Info)
  [info] -> Powertrain & Driveline/3(VehFdbk)
  Vehicle Body 3DOF Dual Track/1 -> [info]
  Lateral and Longitudinal Controller/1(AccelCmd) -> [acc]
  Lateral and Longitudinal Controller/2(DecelCmd) -> [dcc]
  [FwF] -> Vehicle Body 3DOF Dual Track/2
  [FwR] -> Vehicle Body 3DOF Dual Track/3
  [y] -> Mux1/4

== system NN_MPC/Trajectory speed ==
  Demux : Demux  Tag=STV Demux  Outputs=1
      settings: DisplayOption=none
  FromWs : FromWorkspace  Tag=STV FromWs  VariableName=tuvar
      SigBuilderData=|
      | common.afterFinalStr = 'Extrapolate'
      | common.sampleTime = 0
      | dataSet.timeRange = [0 280]
      | dataSet.name = 'Group 1'
      | sbobj.Groups.Name = 'Group 1'
      | sbobj.Groups.Signals.Name = 'Signal 1'
      | sbobj.Groups.Signals.XData = [0 1 2 3 4 5 6 7 8 9 10 11 12 13 14 15 16 17 18 19 20 21 22 23 24 25 26 27 28 29 30 31 32 33 34 35 36 37 38 39 40 41 42 43 44 45 46 47 48 49 50 51 52 53 54 55 56 57 58 59 60 61 62 63 64 65 66 67 68 69 70 71 72 73 74 75 76 77 78 79 80 81 82 83 84 85 86 87 88 89 90 91 92 93 94 95 96 97 98 99 100 101 102 103 104 105 106 107 108 109 110 111 112 113 114 115 116 117 118 119 120 121 122 123 124 125 126 127 128 129 130 131 132 133 134 135 136 137 138 139 140 141 142 143 144 145 146 147 148 149 150 151 152 153 154 155 156 157 158 159 160 161 162 163 164 165 166 167 168 169 170 171 172 173 174 175 176 177 178 179 180 181 182 183 184 185 186 187 188 189 190 191 192 193 194 195 196 197 198 199 200 201 202 203 204 205 206 207 208 209 210 211 212 213 214 215 216 217 218 219 220 221 222 223 224 225 226 227 228 229 230 231 232 233 234 235 236 237 238 239 240 241 242 243 244 245 246 247 248 249 250 251 252 253 254 255 256 257 258 259 260 261 262 263 264 265 266 267 268 269 270 271 272 273 274 275 276 277 278 280]
      | sbobj.Groups.Signals.YData = [0.2 0.6 1 1.4 1.8 2.2 2.6 3 3.4 3.8 4.2 4.6 5 5.4 5.8 6.2 6.6 7 7.4 7.8 8.2 8.6 9 9.4 9.8 10.2 10.6 11 11.4 11.8 12.2 12.6 13 13.4 13.8 14 14.1 14.2 14.3 14.4 14.5 14.6 14.7 14.8 14.9 15 15.1 15.2 15.3 15.4 15.5 15.6 15.7 15.8 15.9 16 16 16 16 16 16 16 16 16 16 16 16 16 16 16 16 16 16 16 16 16 16 16 16 16 16 16 16 16 16 16 16 16 16 16 16 16 16 16 16 16 16 16.2 16.4 16.6 16.8 17 17.2 17.4 17.6 17.8 18 18.2 18.4 18.6 18.8 19 19.2 19.4 19.6 19.8 20 20.2 20.4 20.6 20.8 21 21.2 21.4 21.6 21.8 22 22 22.1 22.2 22.3 22.4 22.5 22.6 22.7 22.8 22.9 23 23.1 23.2 23.3 23.4 23.5 23.6 23.7 23.8 23.9 24 24 24 24 24 24 24 24 24 24 24 24 24 24 24 24 24 24 24 24 24 24 24 24 24 24 24 24 24 24 24 24 24 24 24 24 24 24 24 24 24 24 24 24 24 24 24 24 24 24 24 24 23.8 23.6 23.4 23.2 23 22.8 22.6 22.4 22.2 22 21.8 21.6 21.4 21.2 21 20.8 20.6 20.4 20.2 20 19.8 19.6 19.4 19.2 19 18.8 18.6 18.4 18.2 18 18 17.9 17.8 17.7 17.6 17.5 17.4 17.3 17.2 17.1 17 16.9 16.8 16.7 16.6 16.5 16.4 16.3 16.2 16.1 16 16 16 16 16 16 16 16 16 16 16 16 16 16 16 16 16 16 16 16 16 16 16 16 16 16 16 16 16 16 16]
      | sbobj.Groups.TimeRange = [0 280]
  Signal 1 : Outport  Tag=STV Outport
  wires:
  FromWs/1 -> Demux/1
  Demux/1 -> Signal 1/1

== system NN_MPC/Trajectory speed2 ==
  Demux : Demux  Tag=STV Demux  Outputs=1
      settings: DisplayOption=none
  FromWs : FromWorkspace  Tag=STV FromWs  VariableName=tuvar
      SigBuilderData=|
      | common.afterFinalStr = 'Extrapolate'
      | common.sampleTime = 0
      | dataSet.timeRange = [0 280]
      | dataSet.name = 'Group 1'
      | sbobj.Groups.Name = 'Group 1'
      | sbobj.Groups.Signals.Name = 'Signal 1'
      | sbobj.Groups.Signals.XData = [0 1 2 3 4 5 6 7 8 9 10 11 12 13 14 15 16 17 18 19 20 21 22 23 24 25 26 27 28 29 30 31 32 33 34 35 36 37 38 39 40 41 42 43 44 45 46 47 48 49 50 51 52 53 54 55 56 57 58 59 60 61 62 63 64 65 66 67 68 69 70 71 72 73 74 75 76 77 78 79 80 81 82 83 84 85 86 87 88 89 90 91 92 93 94 95 96 97 98 99 100 101 102 103 104 105 106 107 108 109 110 111 112 113 114 115 116 117 118 119 120 121 122 123 124 125 126 127 128 129 130 131 132 133 134 135 136 137 138 139 140 141 142 143 144 145 146 147 148 149 150 151 152 153 154 155 156 157 158 159 160 161 162 163 164 165 166 167 168 169 170 171 172 173 174 175 176 177 178 179 180 181 182 183 184 185 186 187 188 189 190 191 192 193 194 195 196 197 198 199 200 201 202 203 204 205 206 207 208 209 210 211 212 213 214 215 216 217 218 219 220 221 222 223 224 225 226 227 228 229 230 231 232 233 234 235 236 237 238 239 240 241 242 243 244 245 246 247 248 249 250 251 252 253 254 255 256 257 258 259 260 261 262 263 264 265 266 267 268 269 280]
      | sbobj.Groups.Signals.YData = [0 0.042726450512 0.0954177150571 0.168036698253 0.270540836507 0.413868472125 0.617139522173 0.90342136533 1.29560963215 1.82156382644 2.51957237678 3.42723976466 ... (271 elements, 1x271)]
      | sbobj.Groups.TimeRange = [0 280]
  Signal 1 : Outport  Tag=STV Outport
  wires:
  FromWs/1 -> Demux/1
  Demux/1 -> Signal 1/1

== system NN_MPC/Wind2 ==
  Demux : Demux  Tag=STV Demux  Outputs=1
      settings: DisplayOption=none
  FromWs : FromWorkspace  Tag=STV FromWs  VariableName=tuvar
      SigBuilderData=|
      | common.afterFinalStr = 'Extrapolate'
      | common.sampleTime = 0
      | dataSet.timeRange = [0 28]
      | dataSet.name = 'Group 1'
      | sbobj.Groups.Name = 'Group 1'
      | sbobj.Groups.Signals.Name = 'Signal 2'
      | sbobj.Groups.Signals.XData = [0 0.1 0.2 0.3 0.4 0.5 0.6 0.7 0.8 0.9 1 1.1 1.2 1.3 1.4 1.5 1.6 1.7 1.8 1.9 2 2.1 2.2 2.3 2.4 2.5 2.6 2.7 2.8 2.9 2.9 3 3 3.1 3.2 3.3 3.4 3.5 3.6 3.7 3.8 3.9 4 4.1 4.2 4.3 4.4 4.5 4.6 4.7 4.8 4.9 5 5.1 5.2 5.3 5.4 5.5 5.6 5.7 5.8 5.9 6 6.1 6.2 6.3 6.4 6.5 6.6 6.7 6.8 6.9 7 7.1 7.2 7.3 7.4 7.5 7.6 7.7 7.8 7.9 8 8.1 8.2 8.3 8.4 8.5 8.6 8.7 8.8 8.9 9 9.1 9.2 9.3 9.4 9.5 9.6 9.7 9.8 9.9 10 10.1 10.2 10.3 10.4 10.5 10.6 10.7 10.8 10.9 11 11.1 11.2 11.3 11.4 11.5 11.6 11.7 11.8 11.9 12 12.1 12.2 12.3 12.4 12.5 12.6 12.7 12.8 12.9 13 13.1 13.2 13.3 13.4 13.5 13.6 13.7 13.8 13.9 14 14.1 14.2 14.3 14.4 14.5 14.6 14.7 14.8 14.9 15 15.1 15.2 15.3 15.4 15.5 15.6 15.7 15.8 15.9 16 16.1 16.2 16.3 16.4 16.5 16.6 16.7 16.8 16.9 17 17.1 17.2 17.3 17.4 17.5 17.6 17.7 17.8 17.9 18 18.1 18.2 18.3 18.4 18.5 18.6 18.7 18.8 18.9 19 19.1 19.2 19.3 19.4 19.5 19.6 19.7 19.8 19.9 20 20.1 20.2 20.3 20.4 20.5 20.6 20.7 20.8 20.9 21 21.1 21.2 21.3 21.4 21.5 21.6 21.7 21.8 21.9 22 22.1 22.2 22.3 22.4 22.5 22.6 22.7 22.8 22.9 23 23.1 23.2 23.3 23.4 23.5 23.6 23.7 23.8 23.9 24 24.1 24.2 24.3 24.4 24.5 24.6 24.7 24.8 24.9 25 25.1 25.2 25.3 25.4 25.5 25.6 25.7 25.8 25.9 26 26.1 26.2 26.3 26.4 26.5 26.6 26.7 26.8 28]
      | sbobj.Groups.Signals.YData = [0 0.3 0.6 0.9 1.2 1.5 1.8 2.1 2.4 2.7 3 3.3 4.8 7 12.1 15.2 17.2 17.8 18.3 18.9 19.8 20.8 21.5 21.5 20.8 19.3 17.7 14.8 12 9.6 9.4 8.9 8.7 8.5 8.9 9.2 9.5 9.7 9.7 10 10 10 10 10 10 10 10 10 10 10 10 10 10 10 10 10 10 10 10 10 10 10 10 10 8.6 7.5 7.4 8 9.2 10.8 12.6 13.4 13.6 14 14.4 15 15.6 16 16.5 17.3 17.8 19 19.6 20.2 20.8 21.4 22 22.6 23.2 23.8 24.4 25 25.5 25.9 26.2 26.8 27.2 27.5 27.7 28 28 28 28 28 28 28 28 28 28 28 28 28 28 28 28 28 28 28 28 28 28 28 28 28 28 28 28 28 28 28 28 28.1 28.2 28.2 28.2 27.9 27.4 26.6 26.1 24.7 23.2 20.7 19 18 17.6 17.5 17.2 16.8 16.3 16.3 16.7 16.9 17 16.8 16.7 16.5 16.1 15.6 15.4 14.8 14.2 13.6 13 12.4 11.8 11.2 10.6 10 9.4 8.8 8.2 7.6 7 6.4 5.8 5.2 4.6 4 3.4 2.8 2.2 1.6 1 0.4 -0.2 -0.8 -1.4 -2 -2.4 -2.8 -3.1 -3.5 -3.8 -4.1 -4.1 -4.2 -4.4 -4.4 -4.7 -5 -5 -5 -5 -5 -5 -5 -5 -5 -5 -5 -5 -5 -5.3 -5.4 -5.7 -5.8 -6.1 -6.5 -6.9 -7.5 -8.2 -9.4 -10.6 -11.4 -12.2 -13 -13.8 -14.6 -15.4 -16.2 -17 -17.8 -18.6 -19.4 -19.7 -20 -20.5 -20.9 -21.2 -21.7 -21.8 -22 -22 -22 -22 -22 -22 -22 -22 -22 -22 -22 -22 -22 -22 -22 -22 -22 -22 -22 -22 -22 -22 -22 -22 -22 -22 -22 -22 -22 -22 -22]
      | sbobj.Groups.TimeRange = [0 28]
  Signal 2 : Outport  Tag=STV Outport
  wires:
  FromWs/1 -> Demux/1
  Demux/1 -> Signal 2/1

== system NN_MPC/Wind3 ==
  Demux : Demux  Tag=STV Demux  Outputs=1
      settings: DisplayOption=none
  FromWs : FromWorkspace  Tag=STV FromWs  VariableName=tuvar
      SigBuilderData=|
      | common.afterFinalStr = 'Extrapolate'
      | common.sampleTime = 0
      | dataSet.timeRange = [0 200]
      | dataSet.name = 'Group 1'
      | sbobj.Groups.Name = 'Group 1'
      | sbobj.Groups.Signals.Name = 'Signal 2'
      | sbobj.Groups.Signals.XData = [0 1 2 3 4 5 6 7 8 9 10 11 12 13 14 15 16 17 18 19 20 21 22 23 24 25 26 27 28 29 30 31 32 33 34 35 36 37 38 39 40 41 42 43 44 45 46 47 48 49 50 51 52 53 53 54 55 56 57 58 59 60 61 62 63 64 65 66 67 68 69 70 71 72 73 74 75 76 77 78 79 80 81 82 83 84 85 86 87 88 89 90 91 92 93 94 95 96 97 98 99 100 101 102 103 104 105 106 107 108 109 110 111 112 113 114 115 116 117 118 119 120 121 122 123 124 125 126 127 128 129 130 131 132 133 134 135 136 137 138 139 140 141 142 143 144 145 146 147 148 149 150 151 152 153 154 155 156 157 158 159 160 161 162 163 164 165 166 167 168 169 170 171 172 173 173 174 175 176 177 178 179 180 181 182 183 184 185 186 187 188 189 190 191 192 193 194 195 196 197 198 200]
      | sbobj.Groups.Signals.YData = [5 5.75 6.5 7.25 8 8.75 9.5 10.25 11 11.75 12.5 13.25 14 14.75 15 15.85 16.7 17.55 18 18 18 18 18 18 18 18 18 18 18 18 18 18 18 18 18 18.75 19.5 20.25 21 21.75 22.5 23.25 24 24.75 25.5 26.25 27 27.75 28 28.4 28.5 28.1 27.6 26.7 26.8 25.4 23.9 21.5 20.4 20 20 20 20 20 20 20 20 20 20 20.3 20.8 21.5 21.9 21.2 19.3 19 18.5 18 18.2 20 23.4 26.5 28 28.5 28.3 27.45 26.6 25.75 24.9 24.05 23.2 22.35 21.5 20.65 19.8 18.95 18.1 17.25 16.4 15.55 14.7 13.85 13 12.15 11.3 10.45 10 10 10 10 10 10 10 10 10 10 10 10 10 10 10 10 10 9.6 9.1 8.8 8.4 8.5 8.3 8.08 7.44 6.8 6.16 5.52 4.88 4.24 3.6 2.96 2.32 1.68 1.04 0.4 -0.24 -0.88 -1.52 -2.16 -2.8 -3.44 -4.08 -4.72 -5.36 -6 -6.64 -7.28 -7.92 -8.56 -9.2 -9.84 -10.48 -11 -10.9 -10.7 -10.9 -11.6 -12.3 -13.4 -15.7 -17.4 -18.4 -20.2 -21.3 -22.2 -22.4 -22 -21.6 -21.5 -21.4 -21.1 -21.1 -21.1 -21.7 -23.5 -24.6 -25 -25 -25 -25 -25 -25 -25 -25 -25 -25 -25 -25 -25 -25 -25 -25 -25 -25 -25]
      | sbobj.Groups.TimeRange = [0 200]
  Signal 2 : Outport  Tag=STV Outport
  wires:
  FromWs/1 -> Demux/1
  Demux/1 -> Signal 2/1

== system NN_MPC/concatenate ==
  In1 : Inport
  Matrix Concatenate1 : Concatenate  Mode=Multidimensional array  ConcatenateDimension=2
  Matrix Concatenate2 : Concatenate  Mode=Multidimensional array  ConcatenateDimension=2
  Matrix Concatenate3 : Concatenate  Mode=Multidimensional array  ConcatenateDimension=2
  Transpose : Math  Operator=transpose  SaturateOnIntegerOverflow=on
  Transpose1 : Math  Operator=transpose  SaturateOnIntegerOverflow=on
  mu : Outport
  wires:
  Matrix Concatenate1/1 -> Transpose/1
  In1/1 -> Matrix Concatenate1/2, Matrix Concatenate2/2, Matrix Concatenate2/1, Matrix Concatenate1/1
  Matrix Concatenate3/1 -> mu/1
  Transpose/1 -> Matrix Concatenate3/1
  Matrix Concatenate2/1 -> Transpose1/1
  Transpose1/1 -> Matrix Concatenate3/2

== system NN_MPC/concatenate2 ==
  In1 : Inport
  Matrix Concatenate1 : Concatenate  Mode=Multidimensional array  ConcatenateDimension=2
  Matrix Concatenate2 : Concatenate  Mode=Multidimensional array  ConcatenateDimension=2
  Matrix Concatenate3 : Concatenate  Mode=Multidimensional array  ConcatenateDimension=2
  Transpose : Math  Operator=transpose  SaturateOnIntegerOverflow=on
  Transpose1 : Math  Operator=transpose  SaturateOnIntegerOverflow=on
  mu : Outport
  wires:
  Matrix Concatenate1/1 -> Transpose/1
  In1/1 -> Matrix Concatenate1/2, Matrix Concatenate2/2, Matrix Concatenate2/1, Matrix Concatenate1/1
  Matrix Concatenate3/1 -> mu/1
  Transpose/1 -> Matrix Concatenate3/1
  Matrix Concatenate2/1 -> Transpose1/1
  Transpose1/1 -> Matrix Concatenate3/2

== system NN_MPC/lane change ==
  Demux : Demux  Tag=STV Demux  Outputs=1
      settings: DisplayOption=none
  FromWs : FromWorkspace  Tag=STV FromWs  VariableName=tuvar
      SigBuilderData=|
      | common.afterFinalStr = 'Extrapolate'
      | common.sampleTime = 0
      | dataSet.timeRange = [0 20]
      | dataSet.name = 'Group 1'
      | sbobj.Groups.Name = 'Group 1'
      | sbobj.Groups.Signals.Name = 'Signal 2'
      | sbobj.Groups.Signals.XData = [0 1 2 3 4 5 6 7 8 9 10 11 12 13 14 15 16 17 18 19 20]
      | sbobj.Groups.Signals.YData = [0.05 4.1 8.05 11.6 15.9 18.35 19.15 18.65 16.1 15.05 14.9 16 17.9 20.85 23.45 23.7 19.3 18 16.85 16.55 17.55]
      | sbobj.Groups.TimeRange = [0 20]
  Signal 2 : Outport  Tag=STV Outport
  wires:
  Demux/1 -> Signal 2/1
  FromWs/1 -> Demux/1

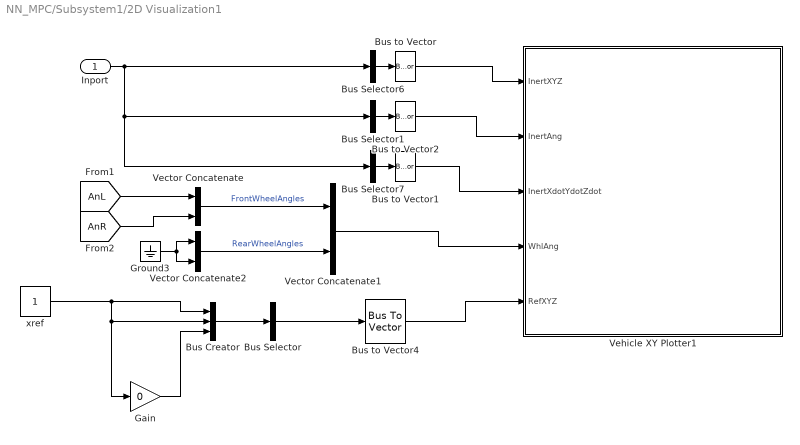
== system NN_MPC/Subsystem1/2D Visualization1 ==
  Inport : Inport
  Bus Creator : BusCreator  Inputs=3
  Bus Selector : BusSelector  OutputSignals=signal1,signal2,signal3  OutputAsBus=on
  Bus Selector1 : BusSelector  OutputSignals=InertFrm.Cg.Ang.phi,InertFrm.Cg.Ang.theta,InertFrm.Cg.Ang.psi  OutputAsBus=on
  Bus Selector6 : BusSelector  OutputSignals=InertFrm.Geom.Disp.X,InertFrm.Geom.Disp.Y,InertFrm.Geom.Disp.Z  OutputAsBus=on
  Bus Selector7 : BusSelector  OutputSignals=InertFrm.Geom.Vel.Xdot,InertFrm.Geom.Vel.Ydot,InertFrm.Geom.Vel.Zdot  OutputAsBus=on
  Bus to Vector{,1..2,4} (4 alike) : BusToVector
  Gain : Gain  Gain=0
  Ground3 : Ground
  Vector Concatenate : Concatenate
  Vector Concatenate1 : Concatenate
  Vector Concatenate2 : Concatenate
  Vehicle XY Plotter1 : Subsystem  mask(Vehicle XY Plotter){extRef=on, extStats=off, extTireF=off, a=2, b=2, w=2, figBorder=10, bufferSize=1024, velNorm=5, tireFNorm=1000, pltDT=0.1}
      mask prompts: extRef "Plot path reference, extRef"; extStats "Display speed, RPM and Gear"; extTireF "Display tire forces"; a "Distance to front axle from CG, a [m]:"; b "Distance to rear axle from CG, b [m]:"; w "Track width, w [m]:"; figBorder "Distance to figure borders, figBorder [m]:"; bufferSize "Path buffer sampe size, bufferSize []:"; velNorm "Velocity vector scaling, velNorm [m*s/m]:"; tireFNorm "Tire force vector scaling, tireFNorm [m/N]:"; pltDT "Plot update rate, pltDT [s]:"
      mask help:
      | This block will display a MATLAB figure which indicates the vehicle path, current position and heading velocity.
      | An optional path reference is also provided.
      mask init:
      | block = gcb;
      | if autoblkschecksimstopped(block)
      |     ParamNames = {'extRef';'extStats';'extTireF';'extTireF'};
      |     PortNames = {'RefXYZ';'Stats';'TireFx';'TireFy'};
      |     for idx=1:length(PortNames)
      |         InportOption  = {'built-in/Ground', [PortNames{idx}, ' Ground'];...
      |             'built-in/Inport',PortNames{idx}};
      |         if ~strcmp(get_param(block,ParamNames{idx}),'on')
      |             NewBlkHdl = autoblksreplaceblock(block, InportOption, 1);
      |             set_param(NewBlkHdl, 'ShowName', 'off');
      |         else
      |             autoblksreplaceblock(block, InportOption, 2);
      |         end
      |     end
      |     InportNames = {'InertXYZ';'InertAng';'InertXdotYdotZdot';'WhlAng';'RefXYZ';'Stats';'TireFx';'TireFy'};
      |     FoundNames = get_param(find_system(block, 'LookUnderMasks', 'all', 'SearchDepth', 1, 'FollowLinks', 'on', 'BlockType', 'Inport'), 'Name');
      |     [~,PortI] = intersect(InportNames, FoundNames);
      |     PortI = sort(PortI);
      |     for idx = 1:length(PortI)
      |         set_param([block, '/', InportNames{PortI(idx)}], 'Port', num2str(idx));
      |     end
      | end
      mask TypeOptions a: Vehicle XY Plotter/a
      mask TypeOptions b: Vehicle XY Plotter/b
      mask TypeOptions w: Vehicle XY Plotter/w
      mask TypeOptions figBorder: Vehicle XY Plotter/figBorder
      mask TypeOptions bufferSize: Vehicle XY Plotter/bufferSize
      mask TypeOptions velNorm: Vehicle XY Plotter/velNorm
      mask TypeOptions tireFNorm: Vehicle XY Plotter/tireFNorm
      mask DialogControl Container3 Prompt: Plot and Display Options
  xref : Constant
  wires:
  Vector Concatenate1/1 -> Vehicle XY Plotter1/4(WhlAng)
  Ground3/1 -> Vector Concatenate2/1, Vector Concatenate2/2
  Bus Selector6/1 -> Bus to Vector/1
  Vector Concatenate/1 -> Vector Concatenate1/1  "FrontWheelAngles"
  [AnL] -> Vector Concatenate/1
  Vector Concatenate2/1 -> Vector Concatenate1/2  "RearWheelAngles"
  Bus Selector7/1 -> Bus to Vector1/1
  Bus to Vector1/1 -> Vehicle XY Plotter1/3(InertXdotYdotZdot)
  Bus to Vector/1 -> Vehicle XY Plotter1/1(InertXYZ)
  Bus to Vector2/1 -> Vehicle XY Plotter1/2(InertAng)
  Bus Selector1/1 -> Bus to Vector2/1
  [AnR] -> Vector Concatenate/2
  Inport/1 -> Bus Selector7/1, Bus Selector1/1, Bus Selector6/1
  Bus to Vector4/1 -> Vehicle XY Plotter1/5(RefXYZ)
  Bus Selector/1 -> Bus to Vector4/1
  xref/1 -> Gain/1, Bus Creator/2, Bus Creator/1
  Gain/1 -> Bus Creator/3
  Bus Creator/1 -> Bus Selector/1

== system NN_MPC/Subsystem1/Bus to Mux1 ==
  Info : Inport
  Bus Selector1 : BusSelector  OutputSignals=InertFrm.Cg.Disp.X,InertFrm.Cg.Disp.Y,InertFrm.Cg.Ang.psi
  Mux : Mux  Inputs=3
  Pose : Outport
  wires:
  Bus Selector1/3 -> Mux/3  "<psi>"
  Bus Selector1/1 -> Mux/1  "<X>"
  Mux/1 -> Pose/1
  Bus Selector1/2 -> Mux/2  "<Y>"
  Info/1 -> Bus Selector1/1

== system NN_MPC/Subsystem1/Concatenate1 ==
  delta : Inport
  Matrix Concatenate : Concatenate
  AnF : Outport  VectorParamsAs1DForOutWhenUnconnected=off
  tag scope: AnL=global, AnR=global
  wires:
  Matrix Concatenate/1 -> AnF/1
  delta/1 -> [AnL], [AnR], Matrix Concatenate/2, Matrix Concatenate/1

== system NN_MPC/Subsystem1/Lateral and Longitudinal Controller1 ==
  VelRef : Inport
  VelFdbk : Inport  Port=2
  Grade : Constant  Value=0
  Longitudinal Driver : autolibshared/Longitudinal Driver  Kp=100  Ki=1  Kff=.1  Kg=0  vnom=9  Kaw=1  tauerr=.01  aMode=2
  Terminator10 : Terminator
  AccelCmd : Outport
  DecelCmd : Outport  Port=2
  wires:
  Longitudinal Driver/3 -> DecelCmd/1
  VelRef/1 -> Longitudinal Driver/1
  VelFdbk/1 -> Longitudinal Driver/2
  Longitudinal Driver/2 -> AccelCmd/1
  Longitudinal Driver/1 -> Terminator10/1
  Grade/1 -> Longitudinal Driver/3

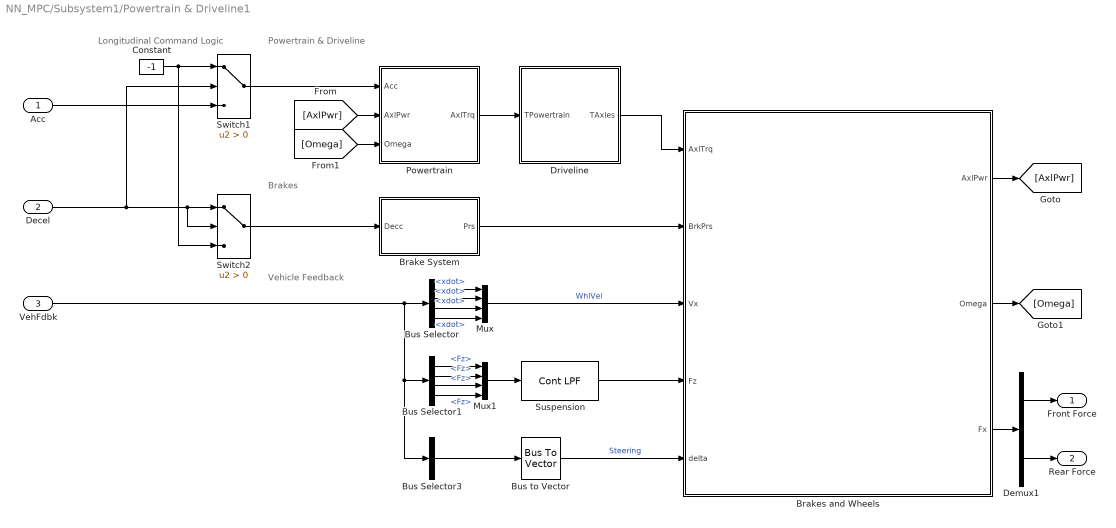
== system NN_MPC/Subsystem1/Powertrain & Driveline1 ==
  note: Vehicle Feedback
  note: Powertrain & Driveline
  note: Brakes
  note: Longitudinal Command Logic
  Acc : Inport
  Decel : Inport  Port=2
  VehFdbk : Inport  Port=3
  Brake System : Subsystem
  Brakes and Wheels : Subsystem  TreatAsAtomicUnit=on
      mask Display: image('vdbslibwhls.png');
  Bus Selector : BusSelector  OutputSignals=BdyFrm.FrntAxl.Lft.Vel.xdot,BdyFrm.FrntAxl.Rght.Vel.xdot,BdyFrm.RearAxl.Lft.Vel.xdot,BdyFrm.RearAxl.Rght.Vel.xdot
  Bus Selector1 : BusSelector  OutputSignals=BdyFrm.Forces.FrntAxl.Lft.Fz,BdyFrm.Forces.FrntAxl.Rght.Fz,BdyFrm.Forces.RearAxl.Lft.Fz,BdyFrm.Forces.RearAxl.Rght.Fz
  Bus Selector3 : BusSelector  OutputSignals=BdyFrm.FrntAxl.Steer.WhlAngFL,BdyFrm.FrntAxl.Steer.WhlAngFR,BdyFrm.RearAxl.Steer.WhlAngRL,BdyFrm.RearAxl.Steer.WhlAngRR  OutputAsBus=on
  Bus to Vector : BusToVector
  Constant : Constant  Value=-1
  Demux1 : Demux  Outputs=[2 2]
  Driveline : Subsystem  Variant=on  VariantControl=Variant1  OverrideUsingVariant=0
  Mux : Mux
  Mux1 : Mux
  Powertrain : Subsystem
  Suspension : autolibutils/Cont LPF  wc=10*pi*2  AbsoluteTolerance=auto  aMode=2
  Switch1 : Switch  Criteria=u2 > Threshold
  Switch2 : Switch  Criteria=u2 > Threshold
  Front Force : Outport  VectorParamsAs1DForOutWhenUnconnected=off
  Rear Force : Outport  Port=2  VectorParamsAs1DForOutWhenUnconnected=off
  wires:
  Brake System/1(Prs) -> Brakes and Wheels/2(BrkPrs)
  Switch2/1 -> Brake System/1(Decc)
  [Omega] -> Powertrain/3(Omega)
  [AxlPwr] -> Powertrain/2(AxlPwr)
  Brakes and Wheels/2(Omega) -> [Omega]
  Powertrain/1(AxlTrq) -> Driveline/1(TPowertrain)
  Switch1/1 -> Powertrain/1(Acc)
  Bus Selector1/4 -> Mux1/4  "<Fz>"
  Bus Selector1/3 -> Mux1/3  "<Fz>"
  Bus Selector1/2 -> Mux1/2  "<Fz>"
  Bus Selector1/1 -> Mux1/1  "<Fz>"
  Bus Selector/4 -> Mux/4  "<xdot>"
  Bus Selector/3 -> Mux/3  "<xdot>"
  Bus Selector/2 -> Mux/2  "<xdot>"
  Bus Selector/1 -> Mux/1  "<xdot>"
  Suspension/1 -> Brakes and Wheels/4(Fz)
  Mux1/1 -> Suspension/1
  Bus to Vector/1 -> Brakes and Wheels/5(delta)  "Steering"
  Bus Selector3/1 -> Bus to Vector/1
  Brakes and Wheels/3(Fx) -> Demux1/1
  Brakes and Wheels/1(AxlPwr) -> [AxlPwr]
  Driveline/1(TAxles) -> Brakes and Wheels/1(AxlTrq)
  Demux1/2 -> Rear Force/1
  Demux1/1 -> Front Force/1
  VehFdbk/1 -> Bus Selector/1, Bus Selector1/1, Bus Selector3/1
  Mux/1 -> Brakes and Wheels/3(Vx)  "WhlVel"
  Constant/1 -> Switch1/1, Switch2/3
  Acc/1 -> Switch1/3
  Decel/1 -> Switch2/1, Switch2/2, Switch1/2

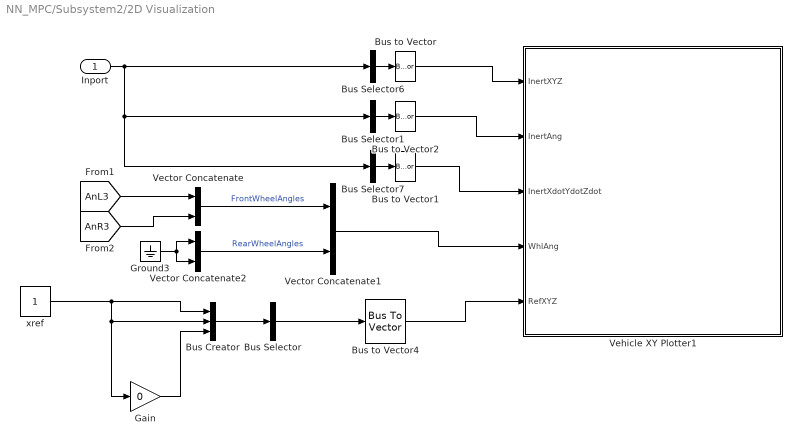
== system NN_MPC/Subsystem2/2D Visualization ==
  Inport : Inport
  Bus Creator : BusCreator  Inputs=3
  Bus Selector : BusSelector  OutputSignals=signal1,signal2,signal3  OutputAsBus=on
  Bus Selector1 : BusSelector  OutputSignals=InertFrm.Cg.Ang.phi,InertFrm.Cg.Ang.theta,InertFrm.Cg.Ang.psi  OutputAsBus=on
  Bus Selector6 : BusSelector  OutputSignals=InertFrm.Geom.Disp.X,InertFrm.Geom.Disp.Y,InertFrm.Geom.Disp.Z  OutputAsBus=on
  Bus Selector7 : BusSelector  OutputSignals=InertFrm.Geom.Vel.Xdot,InertFrm.Geom.Vel.Ydot,InertFrm.Geom.Vel.Zdot  OutputAsBus=on
  Bus to Vector{,1..2,4} (4 alike) : BusToVector
  Gain : Gain  Gain=0
  Ground3 : Ground
  Vector Concatenate : Concatenate
  Vector Concatenate1 : Concatenate
  Vector Concatenate2 : Concatenate
  Vehicle XY Plotter1 : Subsystem  mask(Vehicle XY Plotter){extRef=on, extStats=off, extTireF=off, a=2, b=2, w=2, figBorder=10, bufferSize=1024, velNorm=5, tireFNorm=1000, pltDT=0.1}
      mask prompts: extRef "Plot path reference, extRef"; extStats "Display speed, RPM and Gear"; extTireF "Display tire forces"; a "Distance to front axle from CG, a [m]:"; b "Distance to rear axle from CG, b [m]:"; w "Track width, w [m]:"; figBorder "Distance to figure borders, figBorder [m]:"; bufferSize "Path buffer sampe size, bufferSize []:"; velNorm "Velocity vector scaling, velNorm [m*s/m]:"; tireFNorm "Tire force vector scaling, tireFNorm [m/N]:"; pltDT "Plot update rate, pltDT [s]:"
      mask help:
      | This block will display a MATLAB figure which indicates the vehicle path, current position and heading velocity.
      | An optional path reference is also provided.
      mask init: same as NN_MPC/Subsystem1/2D Visualization1/Vehicle XY Plotter1
      mask TypeOptions a: Vehicle XY Plotter/a
      mask TypeOptions b: Vehicle XY Plotter/b
      mask TypeOptions w: Vehicle XY Plotter/w
      mask TypeOptions figBorder: Vehicle XY Plotter/figBorder
      mask TypeOptions bufferSize: Vehicle XY Plotter/bufferSize
      mask TypeOptions velNorm: Vehicle XY Plotter/velNorm
      mask TypeOptions tireFNorm: Vehicle XY Plotter/tireFNorm
      mask DialogControl Container3 Prompt: Plot and Display Options
  xref : Constant
  wires:
  Vector Concatenate1/1 -> Vehicle XY Plotter1/4(WhlAng)
  Ground3/1 -> Vector Concatenate2/1, Vector Concatenate2/2
  Bus Selector6/1 -> Bus to Vector/1
  Vector Concatenate/1 -> Vector Concatenate1/1  "FrontWheelAngles"
  [AnL3] -> Vector Concatenate/1
  Vector Concatenate2/1 -> Vector Concatenate1/2  "RearWheelAngles"
  Bus Selector7/1 -> Bus to Vector1/1
  Bus to Vector1/1 -> Vehicle XY Plotter1/3(InertXdotYdotZdot)
  Bus to Vector/1 -> Vehicle XY Plotter1/1(InertXYZ)
  Bus to Vector2/1 -> Vehicle XY Plotter1/2(InertAng)
  Bus Selector1/1 -> Bus to Vector2/1
  [AnR3] -> Vector Concatenate/2
  Inport/1 -> Bus Selector7/1, Bus Selector1/1, Bus Selector6/1
  Bus to Vector4/1 -> Vehicle XY Plotter1/5(RefXYZ)
  Bus Selector/1 -> Bus to Vector4/1
  xref/1 -> Gain/1, Bus Creator/2, Bus Creator/1
  Gain/1 -> Bus Creator/3
  Bus Creator/1 -> Bus Selector/1

== system NN_MPC/Subsystem2/Bus to Mux ==
  Info : Inport
  Bus Selector1 : BusSelector  OutputSignals=InertFrm.Cg.Disp.X,InertFrm.Cg.Disp.Y,InertFrm.Cg.Ang.psi
  Mux : Mux  Inputs=3
  Pose : Outport
  wires:
  Bus Selector1/3 -> Mux/3  "<psi>"
  Bus Selector1/1 -> Mux/1  "<X>"
  Mux/1 -> Pose/1
  Bus Selector1/2 -> Mux/2  "<Y>"
  Info/1 -> Bus Selector1/1

== system NN_MPC/Subsystem2/Concatenate ==
  delta : Inport
  Matrix Concatenate : Concatenate
  AnF : Outport  VectorParamsAs1DForOutWhenUnconnected=off
  tag scope: AnL3=global, AnR3=global
  wires:
  Matrix Concatenate/1 -> AnF/1
  delta/1 -> [AnL3], [AnR3], Matrix Concatenate/2, Matrix Concatenate/1

== system NN_MPC/Subsystem2/Lateral and Longitudinal Controller ==
  VelRef : Inport
  VelFdbk : Inport  Port=2
  Grade : Constant  Value=0
  Longitudinal Driver : autolibshared/Longitudinal Driver  Kp=100  Ki=1  Kff=.1  Kg=0  vnom=9  Kaw=1  tauerr=.01  aMode=2
  Terminator10 : Terminator
  AccelCmd : Outport
  DecelCmd : Outport  Port=2
  wires:
  Longitudinal Driver/3 -> DecelCmd/1
  VelRef/1 -> Longitudinal Driver/1
  VelFdbk/1 -> Longitudinal Driver/2
  Longitudinal Driver/2 -> AccelCmd/1
  Longitudinal Driver/1 -> Terminator10/1
  Grade/1 -> Longitudinal Driver/3

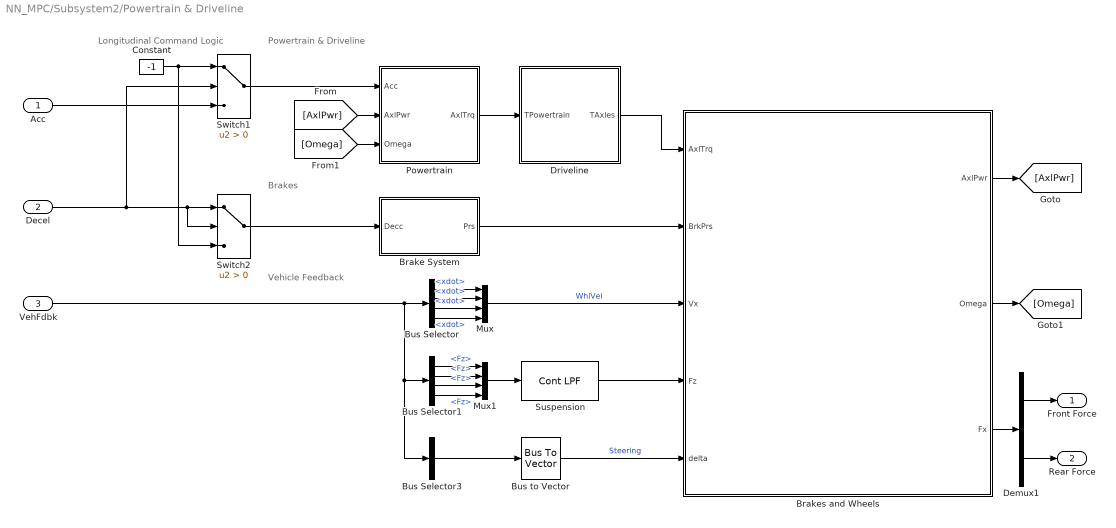
== system NN_MPC/Subsystem2/Powertrain & Driveline ==
  note: Vehicle Feedback
  note: Powertrain & Driveline
  note: Brakes
  note: Longitudinal Command Logic
  Acc : Inport
  Decel : Inport  Port=2
  VehFdbk : Inport  Port=3
  Brake System : Subsystem
  Brakes and Wheels : Subsystem  TreatAsAtomicUnit=on
      mask Display: image('vdbslibwhls.png');
  Bus Selector : BusSelector  OutputSignals=BdyFrm.FrntAxl.Lft.Vel.xdot,BdyFrm.FrntAxl.Rght.Vel.xdot,BdyFrm.RearAxl.Lft.Vel.xdot,BdyFrm.RearAxl.Rght.Vel.xdot
  Bus Selector1 : BusSelector  OutputSignals=BdyFrm.Forces.FrntAxl.Lft.Fz,BdyFrm.Forces.FrntAxl.Rght.Fz,BdyFrm.Forces.RearAxl.Lft.Fz,BdyFrm.Forces.RearAxl.Rght.Fz
  Bus Selector3 : BusSelector  OutputSignals=BdyFrm.FrntAxl.Steer.WhlAngFL,BdyFrm.FrntAxl.Steer.WhlAngFR,BdyFrm.RearAxl.Steer.WhlAngRL,BdyFrm.RearAxl.Steer.WhlAngRR  OutputAsBus=on
  Bus to Vector : BusToVector
  Constant : Constant  Value=-1
  Demux1 : Demux  Outputs=[2 2]
  Driveline : Subsystem  Variant=on  VariantControl=Variant1  OverrideUsingVariant=0
  Mux : Mux
  Mux1 : Mux
  Powertrain : Subsystem
  Suspension : autolibutils/Cont LPF  wc=10*pi*2  AbsoluteTolerance=auto  aMode=2
  Switch1 : Switch  Criteria=u2 > Threshold
  Switch2 : Switch  Criteria=u2 > Threshold
  Front Force : Outport  VectorParamsAs1DForOutWhenUnconnected=off
  Rear Force : Outport  Port=2  VectorParamsAs1DForOutWhenUnconnected=off
  wires:
  Brake System/1(Prs) -> Brakes and Wheels/2(BrkPrs)
  Switch2/1 -> Brake System/1(Decc)
  [Omega] -> Powertrain/3(Omega)
  [AxlPwr] -> Powertrain/2(AxlPwr)
  Brakes and Wheels/2(Omega) -> [Omega]
  Powertrain/1(AxlTrq) -> Driveline/1(TPowertrain)
  Switch1/1 -> Powertrain/1(Acc)
  Bus Selector1/4 -> Mux1/4  "<Fz>"
  Bus Selector1/3 -> Mux1/3  "<Fz>"
  Bus Selector1/2 -> Mux1/2  "<Fz>"
  Bus Selector1/1 -> Mux1/1  "<Fz>"
  Bus Selector/4 -> Mux/4  "<xdot>"
  Bus Selector/3 -> Mux/3  "<xdot>"
  Bus Selector/2 -> Mux/2  "<xdot>"
  Bus Selector/1 -> Mux/1  "<xdot>"
  Suspension/1 -> Brakes and Wheels/4(Fz)
  Mux1/1 -> Suspension/1
  Bus to Vector/1 -> Brakes and Wheels/5(delta)  "Steering"
  Bus Selector3/1 -> Bus to Vector/1
  Brakes and Wheels/3(Fx) -> Demux1/1
  Brakes and Wheels/1(AxlPwr) -> [AxlPwr]
  Driveline/1(TAxles) -> Brakes and Wheels/1(AxlTrq)
  Demux1/2 -> Rear Force/1
  Demux1/1 -> Front Force/1
  VehFdbk/1 -> Bus Selector/1, Bus Selector1/1, Bus Selector3/1
  Mux/1 -> Brakes and Wheels/3(Vx)  "WhlVel"
  Constant/1 -> Switch1/1, Switch2/3
  Acc/1 -> Switch1/3
  Decel/1 -> Switch2/1, Switch2/2, Switch1/2

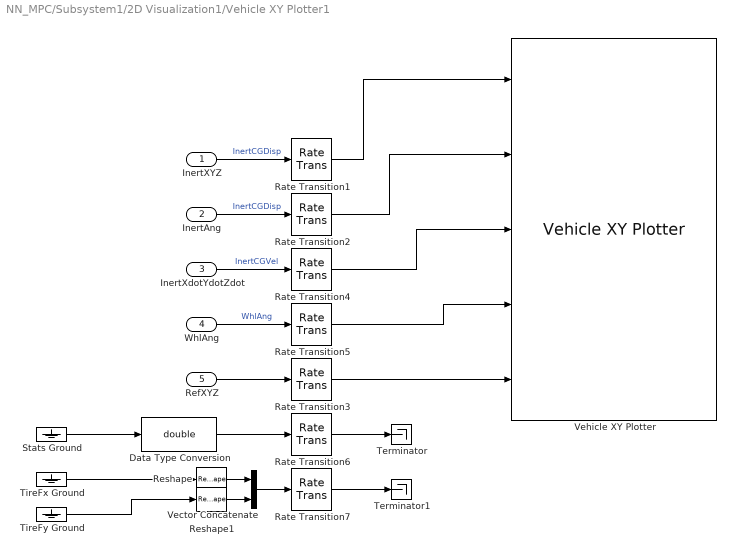
== system NN_MPC/Subsystem1/2D Visualization1/Vehicle XY Plotter1 ==
  InertXYZ : Inport
  InertAng : Inport  Port=2
  InertXdotYdotZdot : Inport  Port=3
  WhlAng : Inport  Port=4
  RefXYZ : Inport  Port=5
  Data Type Conversion : DataTypeConversion  OutDataTypeStr=double
  Rate Transition{1..7} (7 alike) : RateTransition  Deterministic=off  OutPortSampleTime=pltDT
  Reshape : Reshape  OutputDimensionality=Row vector (2-D)
  Reshape1 : Reshape  OutputDimensionality=Row vector (2-D)
  Stats Ground : Ground
  Terminator : Terminator
  Terminator1 : Terminator
  TireFx Ground : Ground
  TireFy Ground : Ground
  Vector Concatenate : Concatenate  Mode=Multidimensional array
  Vehicle XY Plotter : vehdynlibviscommon/Vehicle XY Plotter  w=w  a=a  b=b  figBorder=figBorder  bufferSize=bufferSize
  wires:
  Vector Concatenate/1 -> Rate Transition7/1
  Reshape1/1 -> Vector Concatenate/2
  Reshape/1 -> Vector Concatenate/1
  Rate Transition7/1 -> Terminator1/1
  Data Type Conversion/1 -> Rate Transition6/1
  Rate Transition6/1 -> Terminator/1
  Rate Transition5/1 -> Vehicle XY Plotter/4
  Rate Transition4/1 -> Vehicle XY Plotter/3
  Rate Transition2/1 -> Vehicle XY Plotter/2
  Rate Transition1/1 -> Vehicle XY Plotter/1
  Rate Transition3/1 -> Vehicle XY Plotter/5
  WhlAng/1 -> Rate Transition5/1  "WhlAng"
  InertXYZ/1 -> Rate Transition1/1  "InertCGDisp"
  InertXdotYdotZdot/1 -> Rate Transition4/1  "InertCGVel"
  InertAng/1 -> Rate Transition2/1  "InertCGDisp"
  TireFx Ground/1 -> Reshape/1
  TireFy Ground/1 -> Reshape1/1
  Stats Ground/1 -> Data Type Conversion/1
  RefXYZ/1 -> Rate Transition3/1

== system NN_MPC/Subsystem1/Powertrain & Driveline1/Brake System ==
  Decc : Inport
  Hydraulics : autolibutils/Cont LPF  wc=30*pi*2  AbsoluteTolerance=auto  aMode=2
  Pressure : Gain  Gain=2e7
  Saturation1 : Saturate  UpperLimit=inf  LowerLimit=0  ZeroCross=off
  Selector : Selector  InputPortWidth=1  IndexOptions=Index vector (dialog)  Indices=[1 1 1 1]  OutputSizes=1
  Signal Specification : SignalSpecification  Unit=Pa
  Prs : Outport  VectorParamsAs1DForOutWhenUnconnected=off
  wires:
  Signal Specification/1 -> Prs/1
  Decc/1 -> Saturation1/1
  Selector/1 -> Signal Specification/1
  Saturation1/1 -> Hydraulics/1
  Hydraulics/1 -> Pressure/1
  Pressure/1 -> Selector/1
